simulink model "classicLVariableInductor"  (R2016a)
settings: Solver=VariableStepAuto  StartTime=0  StopTime=simtime  RelTol=1e-4
values from neighbouring files (symbols this model uses):
  a = 1    [ClassicLParameters.m]    (also in Lmeasure.m = (y2-y1)/(x2-x1))
  b = 0    [ClassicLParameters.m]    (also in Lmeasure.m = (y1*x2-x1*y2)/(x2-x1))
  f2 = 2000    [ClassicLParameters.m]
  frad = f*6.283185299990382    (= 628.318529999)    [ClassicLParameters.m]
  ramp = 150*simtime*10    (= 75)    [ClassicLParameters.m]
  Rdrutu = ldrutu*0.0144    (= 0.0012096)    [ClassicLParameters.m]
  vol = 0.2    [ClassicLParameters.m]
libraries: fl_lib x5, nesl_utility x5, simulink x3, dsparch4 x2, elec_lib x1
settings Model: Creator=filipoo  LastModifiedBy=filipoo
settings SolverCC: ZeroCrossAlgorithm=Adaptive

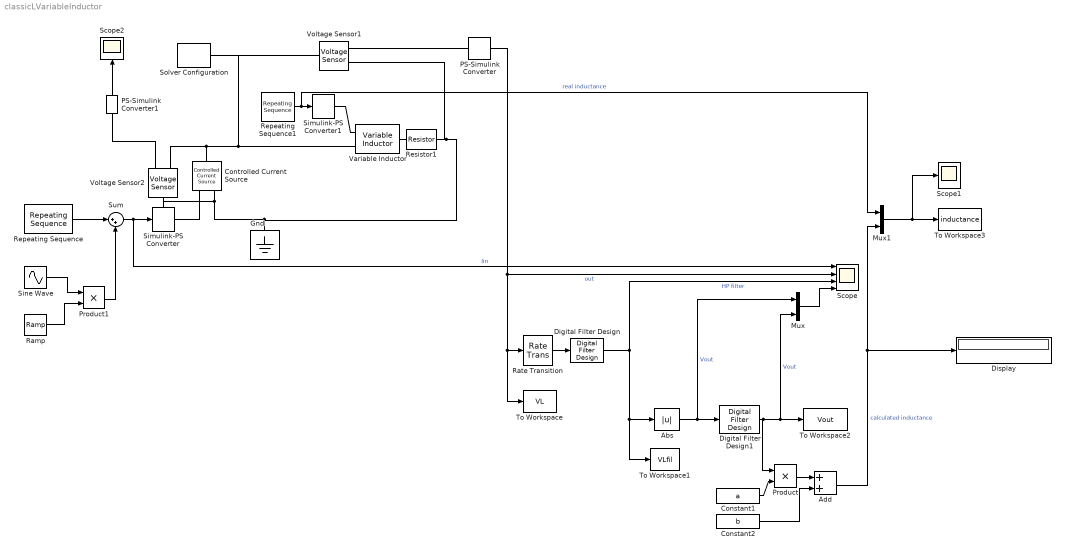
== system classicLVariableInductor ==
  Abs : Abs
  Add : Sum
  Constant1 : Constant  Value=a
  Constant2 : Constant  Value=b
  Controlled Current Source : fl_lib/Electrical/Electrical Sources/Controlled Current Source
  Digital Filter Design : dsparch4/Digital Filter Design  mwdsp_browser_bugfix_var=off
  Digital Filter Design1 : dsparch4/Digital Filter Design  mwdsp_browser_bugfix_var=off
  Display : Display
  Gnd : fl_lib/Electrical/Electrical Elements/Electrical Reference
  Mux : Mux  Inputs=2
  Mux1 : Mux  Inputs=2
  PS-Simulink Converter : nesl_utility/PS-Simulink Converter  PhysicalDomain=network_engine_domain  SubClassName=ps_output  LeftPortType=input  RightPortType=output  PseudoPeriodic=off  Frequencies=[]  Unit=1  AffineConversion=off
  PS-Simulink Converter1 : nesl_utility/PS-Simulink Converter  PhysicalDomain=network_engine_domain  SubClassName=ps_output  LeftPortType=input  RightPortType=output  PseudoPeriodic=off  Frequencies=[]  Unit=1  AffineConversion=off
  Product : Product
  Product1 : Product
  Ramp : simulink/Sources/Ramp  slope=ramp  start=0  X0=0
  Rate Transition : RateTransition  OutPortSampleTime=0.00005
  Repeating Sequence : simulink/Sources/Repeating Sequence  rep_seq_t=[0 0.5 1.5 2.5 3.5 4]*1/(2*f2)  rep_seq_y=[0 1 -1 1 -1 0]*-vol
  Repeating Sequence1 : simulink/Sources/Repeating Sequence  rep_seq_t="[0 0.01 0.011 0.03  0.031]"  rep_seq_y=[0.0013 0.0013 0.0019 0.0019 0.0013]
  Resistor1 : fl_lib/Electrical/Electrical Elements/Resistor  R=Rdrutu Ohm  i_specify=off  i_priority=None  i=0 A  v_specify=off  v_priority=None  v=0 V
  Scope : Scope  NumInputPorts=4
  Scope1 : Scope
  Scope2 : Scope
  Simulink-PS Converter : nesl_utility/Simulink-PS Converter  PhysicalDomain=network_engine_domain  SubClassName=ps_input  LeftPortType=input  RightPortType=output  PseudoPeriodic=off  Frequencies=[]  NoiseDistribution=none  NoiseParameters=[]  Unit=1  AffineConversion=off  InputFiltering=on  SimscapeFilterOrder=2  InputFilterTimeConstant=0.00001  UdotUserProvided=1
  Simulink-PS Converter1 : nesl_utility/Simulink-PS Converter  PhysicalDomain=network_engine_domain  SubClassName=ps_input  LeftPortType=input  RightPortType=output  PseudoPeriodic=off  Frequencies=[]  NoiseDistribution=none  NoiseParameters=[]  Unit=1  AffineConversion=off  InputFiltering=on  SimscapeFilterOrder=2  InputFilterTimeConstant=0.00001  UdotUserProvided=1
  Sine Wave : Sin  Frequency=frad  SampleTime=0
  Solver Configuration : nesl_utility/Solver Configuration  PhysicalDomain=network_engine_domain  SubClassName=solver  LeftPortType=input  RightPortType=generic  Accelerate=off  Tones=[]  Harmonics=[]  SimulateNoise=off  Profile=off  UseLocalSampling=off  EnableSwitchedLinearOptims=on  FrequencyDomain=off  UseCCode=off  RelTol=0.001  AbsTol=1e-06  MinStep=1e-09  ToWorkspace=off  RevertToSquareIcSolve=off  NumHomotopyIterations=100  PhasorMode=off  PhasorModeNumHarmonics=1  OverrideAbsTol=off  DoDC=off  ResidualTolerance=1e-09  UseLocalSolver=off  LocalSolverChoice=NE_BACKWARD_EULER_ADVANCER  LocalSolverSampleTime=0.001  DoFixedCost=off  MaxNonlinIter=3  MaxModeIter=2  LinearAlgebra=Sparse  DelaysMemoryBudget=1024  AutomaticFiltering=on  FilteringTimeConstant=0.001
  Sum : Sum  Inputs=|++
  To Workspace : ToWorkspace  VariableName=VL  SaveFormat=Timeseries  SampleTime=-1
  To Workspace1 : ToWorkspace  VariableName=VLfil  SaveFormat=Timeseries  SampleTime=-1
  To Workspace2 : ToWorkspace  VariableName=Vout  SaveFormat=Timeseries  SampleTime=-1
  To Workspace3 : ToWorkspace  VariableName=inductance  SaveFormat=Timeseries  SampleTime=-1
  Variable Inductor : elec_lib/Passive Devices/Variable Inductor  prm=1  Lmin=1e-6 H  g=1e-9 1/Ohm  i0=0 A  phi0=0 Wb
  Voltage Sensor1 : fl_lib/Electrical/Electrical Sensors/Voltage Sensor
  Voltage Sensor2 : fl_lib/Electrical/Electrical Sensors/Voltage Sensor
  wires:
  PS-Simulink Converter/1 -> Scope/2, To Workspace/1, Rate Transition/1  "out"
  Digital Filter Design/1 -> Scope/3, To Workspace1/1, Abs/1  "HP filter"
  Sum/1 -> Simulink-PS Converter/1, Scope/1  "Iin"
  Rate Transition/1 -> Digital Filter Design/1
  Repeating Sequence/1 -> Sum/1
  Abs/1 -> Digital Filter Design1/1, Mux/1  "Vout"
  Constant1/1 -> Product/2
  Product/1 -> Add/1
  Constant2/1 -> Add/2
  Add/1 -> Display/1, Mux1/2  "calculated inductance"
  Sine Wave/1 -> Product1/1
  Ramp/1 -> Product1/2
  Product1/1 -> Sum/2
  Digital Filter Design1/1 -> Product/1, Mux/2, To Workspace2/1  "Vout"
  Mux/1 -> Scope/4
  PS-Simulink Converter1/1 -> Scope2/1
  Mux1/1 -> Scope1/1, To Workspace3/1
  Repeating Sequence1/1 -> Simulink-PS Converter1/1, Mux1/1  "real inductance"
  connections:
  Simulink-PS Converter/RConn1 -- Controlled Current Source/RConn1
  Controlled Current Source/LConn1 -- Variable Inductor/LConn2 -- Voltage Sensor1/LConn1 -- Solver Configuration/RConn1 -- Voltage Sensor2/RConn2
  Resistor1/RConn1 -- Gnd/LConn1 -- Voltage Sensor2/LConn1 -- Controlled Current Source/RConn2 -- Voltage Sensor1/RConn2
  PS-Simulink Converter/LConn1 -- Voltage Sensor1/RConn1
  PS-Simulink Converter1/LConn1 -- Voltage Sensor2/RConn1
  Variable Inductor/RConn1 -- Resistor1/LConn1
  Simulink-PS Converter1/RConn1 -- Variable Inductor/LConn1
